simulink model "Copy_of_Manuever_1"  (R2023b)
settings: Solver=FixedStepAuto  StartTime=0.0  StopTime=10  RelTol=1e-3  EnableMultiTasking=on
libraries: legoev3lib x7
settings Model: ExtModeBatchMode=on  ExtModeTrigDuration=2  Creator=Krish  LastModifiedBy=Krish
settings SolverCC: PositivePriorityOrder=on  AutoInsertRateTranBlk=on
settings OptimizationCC: EnhancedBackFolding=on  PassReuseOutputArgsAs=Individual arguments  ZeroExternalMemoryAtStartup=off  ZeroInternalMemoryAtStartup=off  MaxStackSize=64  OptimizeBlockOrder=speed  DifferentSizesBufferReuse=on  OptimizationCustomize=off  EfficientTunableParamExpr=on
settings DebuggingCC: ParameterTunabilityLossMsg=error
settings HardwareCC: ProdBitPerPointer=32  ProdBitPerSizeT=32  ProdBitPerPtrDiffT=32  ProdLargestAtomicInteger=Long  ProdWordSize=32  ProdHWDeviceType=ARM Compatible->ARM 9
settings SFSimCC: MATLABDynamicMemAlloc=off
settings RTWCC: Description=Embedded Coder  SystemTargetFile=ert.tlc  HardwareBoard=LEGO MINDSTORMS EV3  TLCOptions="-aInlineSetEventsForThisBaseRateFcn=TLC_FALSE -aSuppressMultiTaskScheduler=TLC_FALSE  -aRateBasedStepFcn=0"  TemplateMakefile=ert_default_tmf  Toolchain=Sourcery G++ Lite v2009q3
settings CodeAppCC: ForceParamTrailComments=on  IgnoreCustomStorageClasses=off  OperatorAnnotations=on  SimulinkDataObjDesc=on  SFDataObjDesc=on  InsertBlockDesc=on
settings ERTTargetCC: SupportContinuousTime=on  SupportVariableSizeSignals=on  ExtModeTransport=2  ExtModeStaticAlloc=on  ExtModeMexFile=ext_xcp  ExtModeIntrfLevel=Level2 - Open

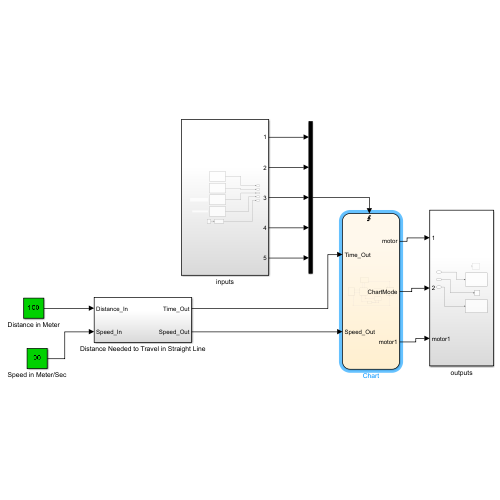
[thumbnail: Simulink's stored preview of the top-level diagram]
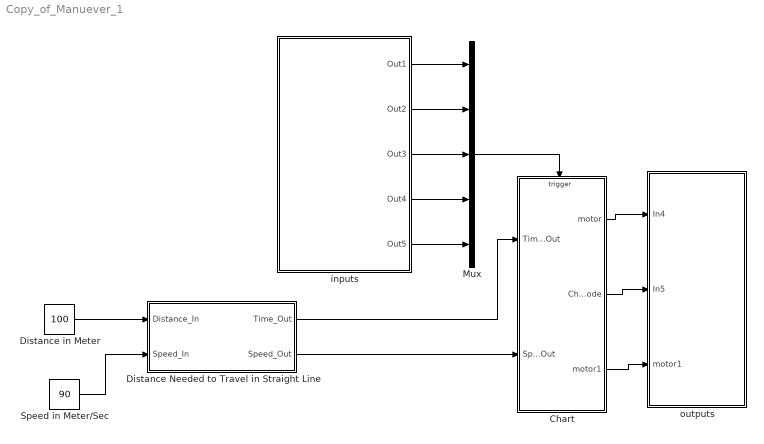
== system Copy_of_Manuever_1 ==
  Chart : Stateflow chart  TreatAsAtomicUnit=on
  Distance Needed to Travel in Straight Line : Subsystem
  Distance in Meter : Constant  Value=100
  Mux : Mux  Inputs=5
  Speed in Meter/Sec : Constant  Value=90
  inputs : Subsystem
  outputs : Subsystem
  wires:
  Mux/1 -> Chart/Trigger
  inputs/1(Out1) -> Mux/1
  inputs/2(Out2) -> Mux/2
  inputs/3(Out3) -> Mux/3
  inputs/4(Out4) -> Mux/4
  inputs/5(Out5) -> Mux/5
  Chart/1(motor) -> outputs/1(In4)
  Chart/2(ChartMode) -> outputs/2(In5)
  Chart/3(motor1) -> outputs/3(motor1)
  Speed in Meter/Sec/1 -> Distance Needed to Travel in Straight Line/2(Speed_In)
  Distance Needed to Travel in Straight Line/1(Time_Out) -> Chart/1(Time_Out)
  Distance in Meter/1 -> Distance Needed to Travel in Straight Line/1(Distance_In)
  Distance Needed to Travel in Straight Line/2(Speed_Out) -> Chart/2(Speed_Out)

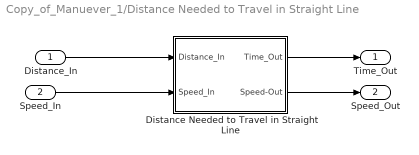
== system Copy_of_Manuever_1/Distance Needed to Travel in Straight Line ==
  Distance_In : Inport
  Speed_In : Inport  Port=2
  Distance Needed to Travel in Straight Line : Subsystem
  Time_Out : Outport
  Speed_Out : Outport  Port=2
  wires:
  Distance Needed to Travel in Straight Line/1(Time_Out) -> Time_Out/1
  Distance_In/1 -> Distance Needed to Travel in Straight Line/1(Distance_In)
  Speed_In/1 -> Distance Needed to Travel in Straight Line/2(Speed_In)
  Distance Needed to Travel in Straight Line/2(Speed-Out) -> Speed_Out/1

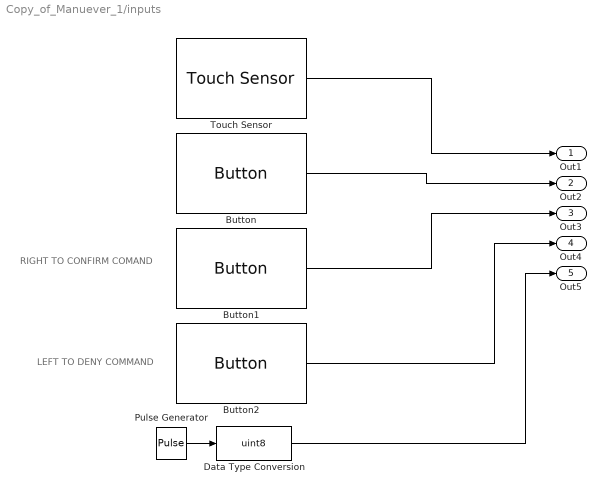
== system Copy_of_Manuever_1/inputs ==
  note: LEFT TO DENY COMMAND
  note: RIGHT TO CONFIRM COMAND
  Button : legoev3lib/Button  buttonType=Center  sampleTime=0.1
  Button1 : legoev3lib/Button  buttonType=Right  sampleTime=0.1
  Button2 : legoev3lib/Button  buttonType=Left  sampleTime=0.1
  Data Type Conversion : DataTypeConversion  OutDataTypeStr=uint8  SaturateOnIntegerOverflow=off  RndMeth=Floor
  Pulse Generator : DiscretePulseGenerator  Period=10  PulseWidth=5  SampleTime=0.1
  Touch Sensor : legoev3lib/Touch Sensor  portNumber=1  sampleTime=0.1
  Out1 : Outport
  Out2 : Outport  Port=2
  Out3 : Outport  Port=3
  Out4 : Outport  Port=4
  Out5 : Outport  Port=5
  wires:
  Pulse Generator/1 -> Data Type Conversion/1
  Button/1 -> Out2/1
  Button2/1 -> Out4/1
  Button1/1 -> Out3/1
  Data Type Conversion/1 -> Out5/1
  Touch Sensor/1 -> Out1/1

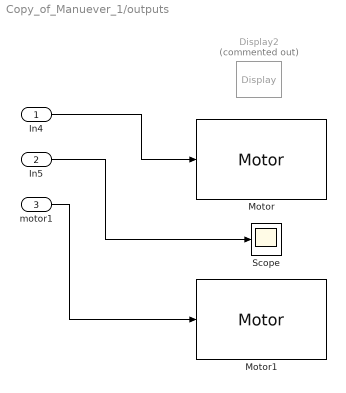
== system Copy_of_Manuever_1/outputs ==
  In4 : Inport
  In5 : Inport  Port=2
  motor1 : Inport  Port=3
  Display2 : legoev3lib/Display  Commented=on  slcdStr=Idle  slcdLine=1  slcdFormat=Decimal
  Motor : legoev3lib/Motor  sportNumber=A  sstopAction=Brake
  Motor1 : legoev3lib/Motor  sportNumber=B  sstopAction=Brake
  Scope : Scope
  wires:
  In4/1 -> Motor/1
  In5/1 -> Scope/1
  motor1/1 -> Motor1/1

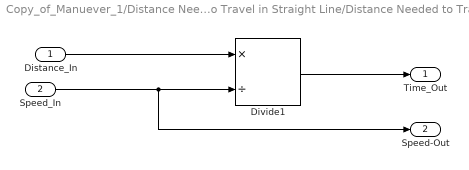
== system Copy_of_Manuever_1/Distance Needed to Travel in Straight Line/Distance Needed to Travel in Straight Line ==
  Distance_In : Inport
  Speed_In : Inport  Port=2
  Divide1 : Product  Inputs=*/
  Time_Out : Outport
  Speed-Out : Outport  Port=2
  wires:
  Speed_In/1 -> Divide1/2, Speed-Out/1
  Distance_In/1 -> Divide1/1
  Divide1/1 -> Time_Out/1

== stateflow chart Copy_of_Manuever_1/Chart ==
  settings: executeAtInitialization=1
  state TurnOffConfirm
    entry:
  state Off
    entry:
    motor=0;
    motor1=0;
    turn_count=0;
  state turn_state
    during:
    motor=0;
    motor1=100;
    turn_count=1+turn_count;
  state On1
    entry:
    motor =Speed_Out;
    motor1=Speed_Out;
  state TurnOnConfirm
  state EmergencySTOP
    entry:
    motor=0;
    motor1=0;
  state mid_state
  TurnOffConfirm -> (junction 129) [order 2] : confirm
  (junction 129) -> Off
  TurnOffConfirm -> On1 [order 1] : deny
  On1 -> TurnOffConfirm [order 3] : Center_btn_pressed
  (default) -> Off
  turn_state -> On1 [order 1] : after(1,sec)
  TurnOnConfirm -> Off [order 2] : deny
  TurnOnConfirm -> On1 [order 1] : confirm
  On1 -> turn_state [order 1] : after(Time_Out,sec)
  Off -> TurnOnConfirm : Center_btn_pressed
  (junction 143) -> Off
  turn_state -> (junction 142) [order 2]
  (junction 113) -> On1
  On1 -> (junction 115) [order 2]
  (junction 115) -> EmergencySTOP : e_btnPressed
  EmergencySTOP -> (junction 128)
  (junction 120) -> EmergencySTOP
  mid_state -> (junction 113) [order 2] : e_btnPressed
  (junction 128) -> mid_state : e_btnPressed
  mid_state -> (junction 120) [order 1] : after(4,sec)
  (junction 142) -> (junction 143) : [turn_count==4]
  data: motor output =0; ChartMode output Enum: ChartModeType; motor1 output; Time_Out input; Speed_Out input; turn_count local =0
  events: e_btnPressed input RISING_EDGE_EVENT; Center_btn_pressed input RISING_EDGE_EVENT; confirm input RISING_EDGE_EVENT; deny input RISING_EDGE_EVENT; clock input RISING_EDGE_EVENT
